simulink model "discrete_smith"  (R2017a)
settings: Solver=VariableStepAuto  StartTime=0.0  StopTime=20.0  RelTol=1e-3
undefined symbols (not defined in the file or in its folder): DiscIntNeverNeededParam
settings Model: Creator=aous  LastModifiedBy=aous

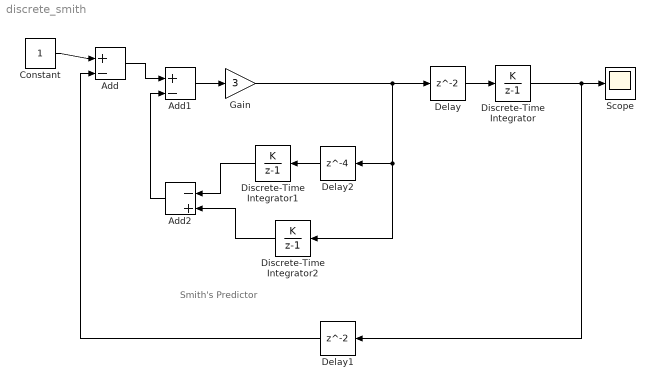
== system discrete_smith ==
  note: Smith's Predictor
  Add : Sum  Inputs=+|-
  Add1 : Sum  Inputs=+|-
  Add2 : Sum  Inputs=-|+
  Constant : Constant
  Delay : Delay  InitialCondition=0
  Delay1 : Delay  InitialCondition=0
  Delay2 : Delay  DelayLength=4  InitialCondition=0
  Discrete-Time Integrator : DiscreteIntegrator  IntegratorMethod=Accumulation: Forward Euler  gainval=0.1  InitialConditionSetting=State (most efficient)  SampleTime=0.1  ICPrevOutput=DiscIntNeverNeededParam  ICPrevScaledInput=DiscIntNeverNeededParam
  Discrete-Time Integrator1 : DiscreteIntegrator  IntegratorMethod=Accumulation: Forward Euler  gainval=0.1  InitialConditionSetting=State (most efficient)  SampleTime=0.1  ICPrevOutput=DiscIntNeverNeededParam  ICPrevScaledInput=DiscIntNeverNeededParam
  Discrete-Time Integrator2 : DiscreteIntegrator  IntegratorMethod=Accumulation: Forward Euler  gainval=0.1  InitialConditionSetting=State (most efficient)  SampleTime=0.1  ICPrevOutput=DiscIntNeverNeededParam  ICPrevScaledInput=DiscIntNeverNeededParam
  Gain : Gain  Gain=3
  Scope : Scope
  wires:
  Gain/1 -> Delay2/1, Discrete-Time Integrator2/1, Delay/1
  Constant/1 -> Add/1
  Add/1 -> Add1/1
  Discrete-Time Integrator/1 -> Scope/1, Delay1/1
  Delay/1 -> Discrete-Time Integrator/1
  Delay1/1 -> Add/2
  Add1/1 -> Gain/1
  Delay2/1 -> Discrete-Time Integrator1/1
  Discrete-Time Integrator1/1 -> Add2/1
  Discrete-Time Integrator2/1 -> Add2/2
  Add2/1 -> Add1/2
